simulink model "sistemaLinearOrdem3"  (R2019a)
settings: Solver=VariableStepAuto  StartTime=0.0  StopTime=10.0  MaxStep=0.001  RelTol=1e-3
values from neighbouring files (symbols this model uses):
  p = linspace(0.1,1.2,50)    [ex_1.m]
settings Model: Creator=thiag  LastModifiedBy=thiag

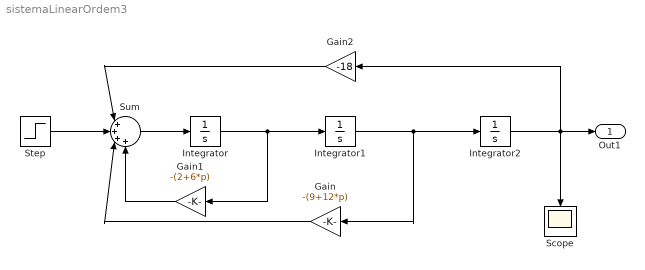
== system sistemaLinearOrdem3 ==
  Gain : Gain  Gain=-(9+12*p)
  Gain1 : Gain  Gain=-(2+6*p)
  Gain2 : Gain  Gain=-18
  Integrator : Integrator
  Integrator1 : Integrator
  Integrator2 : Integrator
  Scope : Scope
  Step : Step  Before=18  After=18  SampleTime=0
  Sum : Sum  Inputs=|++++
  Out1 : Outport
  wires:
  Step/1 -> Sum/2
  Sum/1 -> Integrator/1
  Integrator/1 -> Gain1/1, Integrator1/1
  Integrator1/1 -> Gain/1, Integrator2/1
  Integrator2/1 -> Gain2/1, Scope/1, Out1/1
  Gain/1 -> Sum/3
  Gain1/1 -> Sum/4
  Gain2/1 -> Sum/1
